simulink model "HILFT_WSHP_MPC_2020a"  (R2020a)
settings: Solver=FixedStepAuto  StartTime=20476800  StopTime=20476800  FixedStep=60  RelTol=1e-3
settings Model: Creator=caleb  LastModifiedBy=yl3328
settings DataIOCC: SaveState=on  LoggingToFile=on
settings DebuggingCC: UnconnectedInputMsg=none  UnconnectedOutputMsg=none  UnconnectedLineMsg=none  SFMachineParentedDataDiag=error
settings ModelReferenceCC: EnableRefExpFcnMdlSchedulingChecks=off
settings RTWCC: Description=Generic Real-Time Target

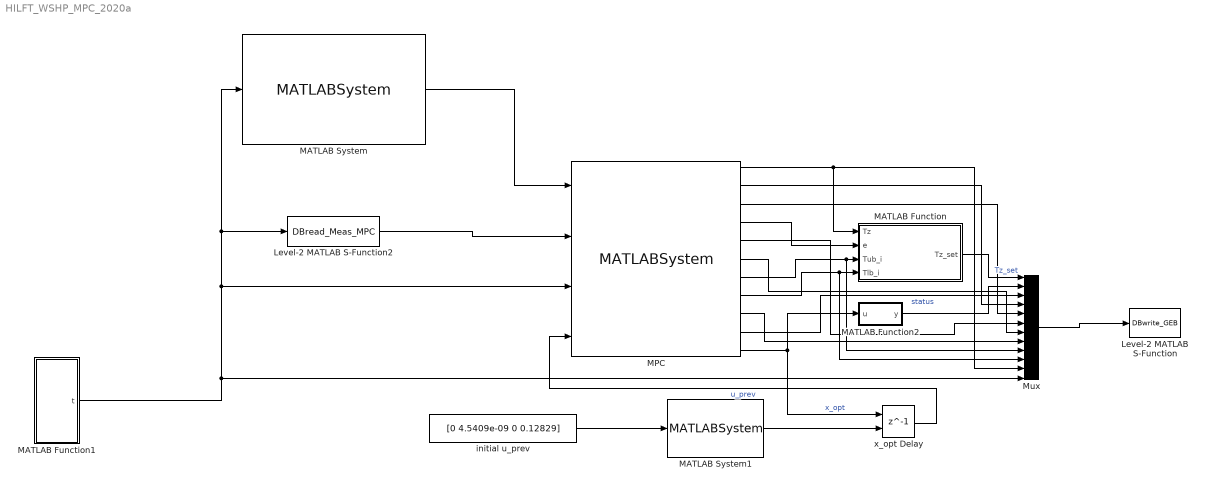
== system HILFT_WSHP_MPC_2020a ==
  Level-2 MATLAB S-Function : M-S-Function  FunctionName=DBwrite_GEB
  Level-2 MATLAB S-Function2 : M-S-Function  FunctionName=DBread_Meas_MPC
  MATLAB Function : MATLAB Function  TreatAsAtomicUnit=on
  MATLAB Function1 : MATLAB Function  TreatAsAtomicUnit=on
  MATLAB Function2 : MATLAB Function  TreatAsAtomicUnit=on
  MATLAB System : MATLABSystem  System=Forecast_Block  PH=16  dt=900  SimulateUsing=Interpreted execution
      mask Type: Forecast_Block
      mask Display:
      | disp('Forecast_Block');
      | port_label('input',1,'time');
      | port_label('output',1,'predictors');
  MATLAB System1 : MATLABSystem  System=repmat_func  PH=16  SimulateUsing=Interpreted execution
      mask Type: repmat_func
      mask Display:
      | disp('repmat_func');
      | port_label('input',1,'u');
      | port_label('output',1,'y');
  MPC : MATLABSystem  System=WSHP_MPC  PH=16  CH=1  dt=900  occ_start=6  occ_end=22  w="[1  1000     0]"  u_lb="[0  0  0  0]"  u_ub="[1          0.1           20            5]"  Tz_lb_unocc=12  Tz_ub_unocc=30  Tz_lb_occ=20  Tz_ub_occ=26.3889  t_start=237*24*3600  price_tou="[0.00746     0.00746     0.00746     0.00746     0.00746     0.00746     0.00746     0.00746     0.00746     0.00746     0.00746     0.00746     0.00746     0.01692     0.01692     0.01692     0.01692     0.01692     0.00746     0.00746     0.00746     0.00746     0.00746     0.00746]"  Tb=17.8  dep=112.8  SimulateUsing=Interpreted execution
      mask Type: WSHP_MPC
      mask Display:
      | disp('WSHP_MPC');
      | port_label('input',1,'predictors');
      | port_label('input',2,'state');
      | port_label('input',3,'time');
      | port_label('input',4,'u_prev');
      | port_label('output',1,'Tz_opt');
      | port_label('output',2,'T2_opt');
      | port_label('output',3,'y_opt');
      | port_label('output',4,'e_opt');
      | port_label('output',5,'q_opt');
      | port_label('output',6,'p_opt');
      | port_label('output',7,'Tub_i');
      | port_label('output',8,'Tlb_i');
      | port_label('output',9,'price');
      | port_label('output',10,'status');
      | port_label('output',11,'x_opt');
  Mux : Mux  Inputs=12
  initial u_prev : Constant  Value="[0  4.5409e-09           0     0.12829]"  VectorParams1D=off
  x_opt Delay : Delay  DelayLength=1  InitialConditionSource=Input port  SampleTime=900
      settings: InputPortMap=u0,p4
  wires:
  MATLAB Function1/1(t) -> MPC/3, Level-2 MATLAB S-Function2/1, MATLAB System/1, Mux/12
  MATLAB System/1 -> MPC/1
  x_opt Delay/1 -> MPC/4  "u_prev"
  initial u_prev/1 -> MATLAB System1/1
  MATLAB System1/1 -> x_opt Delay/2
  Level-2 MATLAB S-Function2/1 -> MPC/2
  MPC/1 -> Mux/11, MATLAB Function/1(Tz)
  MATLAB Function/1(Tz_set) -> Mux/1  "Tz_set"
  Mux/1 -> Level-2 MATLAB S-Function/1
  MATLAB Function2/1(y) -> Mux/2
  MPC/4 -> MATLAB Function/2(e)
  MPC/7 -> Mux/9, MATLAB Function/3(Tub_i)
  MPC/8 -> MATLAB Function/4(Tlb_i), Mux/10
  MPC/10 -> Mux/3  "status"
  MPC/11 -> x_opt Delay/1, MATLAB Function2/1(u)  "x_opt"
  MPC/2 -> Mux/4
  MPC/3 -> Mux/5
  MPC/5 -> Mux/6
  MPC/6 -> Mux/7
  MPC/9 -> Mux/8

== matlab function HILFT_WSHP_MPC_2020a/MATLAB Function2 ==
  data: u input; y output
function y = fcn(u)
y = u(1:4);

== matlab function HILFT_WSHP_MPC_2020a/MATLAB Function ==
  data: Tz input; e input; Tz_set output; Tub_i input; Tlb_i input
function Tz_set = fcn(Tz,e,Tub_i,Tlb_i)
Tz_set=min(Tub_i+e,Tz);
Tz_set=max(Tz_set,Tlb_i-e);

== matlab function HILFT_WSHP_MPC_2020a/MATLAB Function1 ==
  data: t output
function t  = fcn
coder.extrinsic('xlsread');
T=0;
[T] = xlsread('Time.xlsx', 1,'B1');
t=0;
t=T+15*60; %237*86400+645*60;
